simulink model "Servo_Model"  (R2019b)
settings: Solver=VariableStepAuto  StartTime=0.0  StopTime=100  RelTol=1e-3
values from neighbouring files (symbols this model uses):
  B = 0.1    [Servo_Param (1).m]    (also in servoParameters.m)
  Jd = 0.1    [Servo_Param (1).m]    (also in servoParameters.m = 1)
  Km = 1    [Servo_Param (1).m]    (also in servoParameters.m)
libraries: fl_lib x16, ee_lib x8, nesl_utility x8, fl_ps_legacy_lib x2, simulink x2
settings Model: Creator=covasanvictor  LastModifiedBy=covasanvictor
settings SolverCC: ZeroCrossAlgorithm=Adaptive
settings DataIOCC: Refine=100
settings DebuggingCC: MaskedZcDiagnostic=none  IgnoredZcDiagnostic=none
settings SFSimCC: CustomCodeUndefinedFunction=UseInterfaceOnly

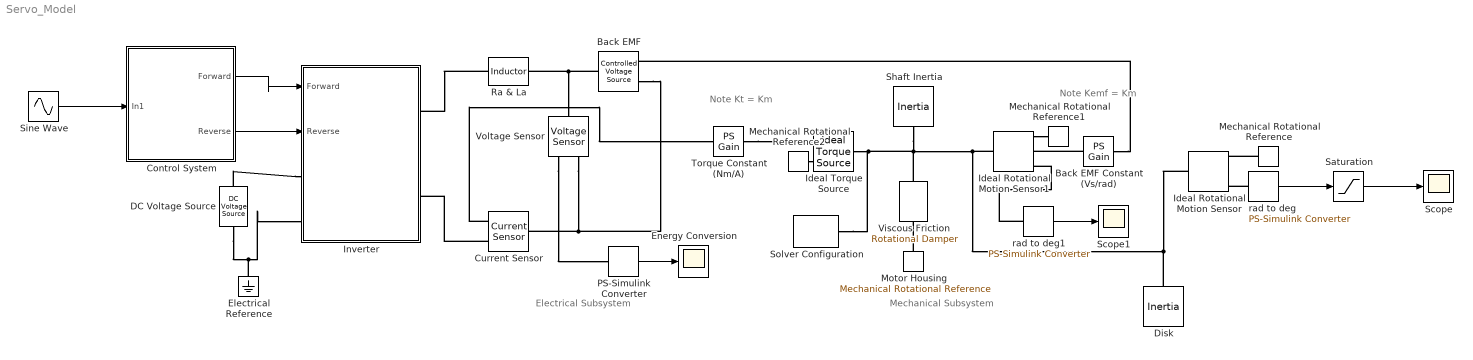
== system Servo_Model ==
  note: Mechanical
      | Subsystem
  note: Note
      | Kemf = Km
  note: Electrical
      | Subsystem
  note: Note
      | Kt = Km
  Back EMF : fl_lib/Electrical/Electrical Sources/Controlled Voltage Source
  Back EMF Constant (Vs/rad) : fl_ps_legacy_lib/Legacy Physical Signals/Functions/PS Gain  gain=Km
      settings: SourceProductName=Simscape
  Control System : Subsystem
  Current Sensor : fl_lib/Electrical/Electrical Sensors/Current Sensor
  DC Voltage Source : fl_lib/Electrical/Electrical Sources/DC Voltage Source  v0=6.2 V
  Disk : fl_lib/Mechanical/Rotational Elements/Inertia  inertia=Jd*21 kg*m^2  w_specify=off  w_priority=Low  w=0 rad/s  w_nominal_specify=off  w_nominal_unit=rad/s  w_nominal_value=1  t_specify=off  t_priority=None  t=0 N*m  t_nominal_specify=off  t_nominal_unit=N*m  t_nominal_value=1
  Electrical Reference : fl_lib/Electrical/Electrical Elements/Electrical Reference
  Energy Conversion : Scope
  Ideal Rotational Motion Sensor : fl_lib/Mechanical/Mechanical Sensors/Ideal Rotational Motion Sensor  offset=90 deg
  Ideal Rotational Motion Sensor1 : fl_lib/Mechanical/Mechanical Sensors/Ideal Rotational Motion Sensor  offset=90 deg
  Ideal Torque Source : fl_lib/Mechanical/Mechanical Sources/Ideal Torque Source
  Inverter : Subsystem
  Mechanical Rotational Reference : fl_lib/Mechanical/Rotational Elements/Mechanical Rotational Reference
  Mechanical Rotational Reference1 : fl_lib/Mechanical/Rotational Elements/Mechanical Rotational Reference
  Mechanical Rotational Reference2 : fl_lib/Mechanical/Rotational Elements/Mechanical Rotational Reference
  Motor Housing : fl_lib/Mechanical/Rotational Elements/Mechanical Rotational Reference
  PS-Simulink Converter : nesl_utility/PS-Simulink Converter  PhysicalDomain=network_engine_domain  SubClassName=ps_output  LeftPortType=input  RightPortType=output  PseudoPeriodic=off  Frequencies=[]  Unit=1  AffineConversion=off
  Ra & La : fl_lib/Electrical/Electrical Elements/Inductor  l=La H  r=Ra Ohm  g=0 1/Ohm  i_specify=off  i_priority=None  i=0 A  i_nominal_specify=off  i_nominal_unit=A  i_nominal_value=1  v_specify=off  v_priority=None  v=0 V  v_nominal_specify=off  v_nominal_unit=V  v_nominal_value=1  i_L_specify=off  i_L_priority=High  i_L=0 A  i_L_nominal_specify=off  i_L_nominal_unit=A  i_L_nominal_value=1
  Saturation : Saturate  UpperLimit=180  LowerLimit=-180
  Scope : Scope
  Scope1 : Scope
  Shaft Inertia : fl_lib/Mechanical/Rotational Elements/Inertia  inertia=J kg*m^2  w_specify=off  w_priority=High  w=0 rad/s  w_nominal_specify=off  w_nominal_unit=rad/s  w_nominal_value=1  t_specify=off  t_priority=None  t=0 N*m  t_nominal_specify=off  t_nominal_unit=N*m  t_nominal_value=1
  Sine Wave : Sin  Amplitude=70  Bias=100  Frequency=0.5  SampleTime=0
  Solver Configuration : nesl_utility/Solver Configuration  PhysicalDomain=network_engine_domain  SubClassName=solver  LeftPortType=input  RightPortType=generic  Tones=[]  Harmonics=[]  SimulateNoise=off  Profile=off  UseLocalSampling=off  EnableSwitchedLinearOptims=on  FrequencyDomain=off  UseCCode=off  RelTol=0.001  AbsTol=1e-06  MinStep=1e-09  ToWorkspace=off  RevertToSquareIcSolve=off  NumHomotopyIterations=100  PhasorMode=off  PhasorModeNumHarmonics=1  DoDC=off  ResidualTolerance=1e-9  UseLocalSolver=off  LocalSolverChoice=NE_BACKWARD_EULER_ADVANCER  LocalSolverSampleTime=.001  DoFixedCost=off  MaxNonlinIter=3  MaxModeIter=2  LinearAlgebra=Sparse  EquationFormulation=NE_TIME_EF  DelaysMemoryBudget=1024  AutomaticFiltering=on  FilteringTimeConstant=0.001  PartitionStorageMethod=AS_NEEDED  PartitionMemoryBudget=1024  PartitionMethod=FAST
  Torque Constant (Nm/A) : fl_ps_legacy_lib/Legacy Physical Signals/Functions/PS Gain  gain=Km
      settings: SourceProductName=Simscape
  Viscous Friction : fl_lib/Mechanical/Rotational Elements/Rotational Damper  D=B N*m/(rad/s)  w_specify=off  w_priority=None  w=0 rad/s  w_nominal_specify=off  w_nominal_unit=rad/s  w_nominal_value=1  t_specify=off  t_priority=None  t=0 N*m  t_nominal_specify=off  t_nominal_unit=N*m  t_nominal_value=1
  Voltage Sensor : fl_lib/Electrical/Electrical Sensors/Voltage Sensor
  rad to deg : nesl_utility/PS-Simulink Converter  PhysicalDomain=network_engine_domain  SubClassName=ps_output  LeftPortType=input  RightPortType=output  PseudoPeriodic=off  Frequencies=[]  Unit=deg  AffineConversion=off
  rad to deg1 : nesl_utility/PS-Simulink Converter  PhysicalDomain=network_engine_domain  SubClassName=ps_output  LeftPortType=input  RightPortType=output  PseudoPeriodic=off  Frequencies=[]  Unit=deg  AffineConversion=off
  wires:
  PS-Simulink Converter/1 -> Energy Conversion/1
  rad to deg1/1 -> Scope1/1
  rad to deg/1 -> Saturation/1
  Saturation/1 -> Scope/1
  Control System/1(Forward) -> Inverter/1(Forward)
  Control System/2(Reverse) -> Inverter/2(Reverse)
  Sine Wave/1 -> Control System/1(In1)
  connections:
  Solver Configuration/RConn1 -- Viscous Friction/RConn1 -- Ideal Rotational Motion Sensor/LConn1 -- Disk/LConn1 -- Ideal Rotational Motion Sensor1/LConn1 -- Shaft Inertia/LConn1 -- Ideal Torque Source/LConn1
  rad to deg/LConn1 -- Ideal Rotational Motion Sensor/RConn3
  Mechanical Rotational Reference/LConn1 -- Ideal Rotational Motion Sensor/RConn1
  Voltage Sensor/RConn2 -- Current Sensor/LConn1 -- Back EMF/RConn2
  Ra & La/RConn1 -- Back EMF/LConn1 -- Voltage Sensor/LConn1
  Current Sensor/RConn1 -- Torque Constant (Nm/A)/LConn1
  Mechanical Rotational Reference2/LConn1 -- Ideal Torque Source/RConn2
  Voltage Sensor/RConn1 -- PS-Simulink Converter/LConn1
  Torque Constant (Nm/A)/RConn1 -- Ideal Torque Source/RConn1
  Back EMF Constant (Vs/rad)/RConn1 -- Back EMF/RConn1
  Motor Housing/LConn1 -- Viscous Friction/LConn1
  Ideal Rotational Motion Sensor1/RConn1 -- Mechanical Rotational Reference1/LConn1
  Back EMF Constant (Vs/rad)/LConn1 -- Ideal Rotational Motion Sensor1/RConn2
  rad to deg1/LConn1 -- Ideal Rotational Motion Sensor1/RConn3
  DC Voltage Source/RConn1 -- Electrical Reference/LConn1 -- Inverter/LConn2
  Ra & La/LConn1 -- Inverter/RConn1
  DC Voltage Source/LConn1 -- Inverter/LConn1
  Current Sensor/RConn2 -- Inverter/RConn2

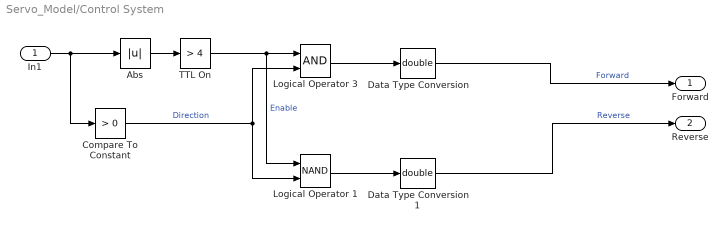
== system Servo_Model/Control System ==
  In1 : Inport
  Abs : Abs
  Compare To Constant : simulink/Logic and Bit Operations/Compare To Constant  relop=>  const=0  OutDataTypeStr=boolean  ZeroCross=off
  Data Type Conversion : DataTypeConversion  OutDataTypeStr=double
  Data Type Conversion1 : DataTypeConversion  OutDataTypeStr=double
  Logical Operator 1 : Logic  Operator=NAND  AllPortsSameDT=off  OutDataTypeStr=boolean
  Logical Operator 3 : Logic  AllPortsSameDT=off  OutDataTypeStr=boolean
  TTL On : simulink/Logic and Bit Operations/Compare To Constant  relop=>  const=4  OutDataTypeStr=boolean  ZeroCross=off
  Forward : Outport  VectorParamsAs1DForOutWhenUnconnected=off
  Reverse : Outport  Port=2  VectorParamsAs1DForOutWhenUnconnected=off
  wires:
  TTL On/1 -> Logical Operator 3/1, Logical Operator 1/1  "Enable"
  Compare To Constant/1 -> Logical Operator 1/2, Logical Operator 3/2  "Direction"
  Logical Operator 3/1 -> Data Type Conversion/1
  Data Type Conversion1/1 -> Reverse/1  "Reverse"
  Logical Operator 1/1 -> Data Type Conversion1/1
  Data Type Conversion/1 -> Forward/1  "Forward"
  In1/1 -> Abs/1, Compare To Constant/1
  Abs/1 -> TTL On/1

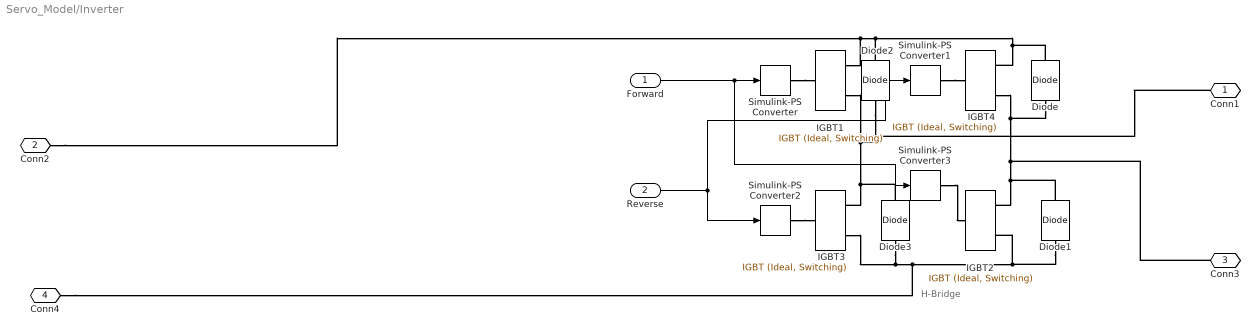
== system Servo_Model/Inverter ==
  note: H-Bridge
  Forward : Inport
  Reverse : Inport  Port=2
  Diode{,1..3} (4 alike) : ee_lib/Semiconductors & Converters/Diode  ModelType=ee.enum.diode.modelType.pwl  Vf=0.6 V  Ron=0.3 Ohm  Goff=1e-8 S  prmExp=ee.enum.diode.expParam.useTwo  I12=[.0137, .545] A  V12=[.6, .7] V  IS=1e-12 A  ec=1  I1=0.0137 A  V1=0.6 V  RS=0 Ohm  Tmeas=25 degC  N_series=1  N_parallel=1  Rz=0.3 Ohm  BV=inf V  C_param=ee.enum.diode.capParam.fixed  CJ=5 pF  CJ0=5 pF  VJ=1 V  Mgrad=0.5  Vvec=[.1, 10, 100] V  Cvec=[3.5, 1, .4] pF  FC=0.5  Q_param=ee.enum.diode.recoveryParam.off  iRM=-7.15 A  iF=4 A  didt=-750 A/us  trr_factor=3  trr=115 ns  Qrr=1500 s*uA  TT=50 ns  tau=100 ns  T_param=ee.enum.diode.temperatureParam.off  IS_T2=1.25e-7 A  I1_T2=0.245 A  V1_T2=0.5 V  Tmeas2=125 degC  EG_param=ee.enum.diode.egapParam.material_si  EG=1.11 eV  XTI_param=ee.enum.diode.xtiParam.pn  XTI=3  dBVdT=0 V/K  Tdevice=25 degC  i_specify=off  i_priority=None  i=0 A  i_nominal_specify=off  i_nominal_unit=A  i_nominal_value=1  v_specify=off  v_priority=None  v=0 V  v_nominal_specify=off  v_nominal_unit=V  v_nominal_value=1  i_capacitor_specify=off  i_capacitor_priority=None  i_capacitor=0 A  i_capacitor_nominal_specify=off  i_capacitor_nominal_unit=A  i_capacitor_nominal_value=1  v_capacitor_specify=off  v_capacitor_priority=None  v_capacitor=0 V  v_capacitor_nominal_specify=off  v_capacitor_nominal_unit=V  v_capacitor_nominal_value=1  power_dissipated_specify=off  power_dissipated_priority=None  power_dissipated=0 W  power_dissipated_nominal_specify=off  power_dissipated_nominal_unit=W  power_dissipated_nominal_value=1  thermal_network_parameterization=ee.enum.thermalNetworkTopology.cauer  Rth=[0, 10] K/W  Rth_Foster=[4, 6] K/W  thermal_mass_parameterization=ee.enum.thermalNetwork.timeconstant  thermal_mass=[0, 1] J/K  thermal_mass_Foster=[1.5, 3] J/K  thermal_time_constant=[0, 10] s  thermal_time_constant_Foster=[6, 18] s  thermal_mass_initial_temperatures=[25, 25] degC
      settings: SourceProductName=Simscape Electrical
  IGBT{1..4} (4 alike) : ee_lib/Semiconductors & Converters/IGBT (Ideal, Switching)  Vf=1 V  Ron=0.001 Ohm  Goff=1e-5 1/Ohm  Vth=0.5 V  diode_param=1  diode_Vf=0.8 V  diode_Ron=0.001 Ohm  diode_Goff=1e-5 1/Ohm  diode_C=5e-8 F  diode_iRM=-235 A  diode_iF=300 A  diode_idot=-50 A/us  diode_trr_param=1  diode_trr_factor=3  diode_trr=15 us  diode_Qrr=1.5e+3 s*uA  thermal_loss_option=2  Voff=300 V  Tau=1e-4 s  Tj=[298.15, 398.15] K  Iout_scalar=600 A  Eon_scalar=22.86e-3 J  Eoff_scalar=17.14e-3 J  Von_scalar=2.7 V  Iout_data=[0, 10, 50, 100, 200, 400, 600] A  Eon_data=[0, .29, 1.43, 2.86, 5.71, 13.14, 22.86; 0, .57, 2.63, 5.14, 10.29, 20.57, 30.29] * 1e-3 J  Eoff_data=[0, .21, 1.07, 2.14, 4.29, 9.86, 17.14; 0, .43, 1.97, 3.86, 7.71, 15.43, 22.71] * 1e-3 J  Von_data=[0, 1.1, 1.3, 1.45, 1.75, 2.25, 2.7; 0, 1, 1.15, 1.35, 1.7, 2.35, 3] V
      settings: SourceProductName=Simscape Electrical
  Simulink-PS Converter{,1..3} (4 alike) : nesl_utility/Simulink-PS Converter  PhysicalDomain=network_engine_domain  SubClassName=ps_input  LeftPortType=input  RightPortType=output  PseudoPeriodic=off  Frequencies=[]  NoiseDistribution=none  NoiseParameters=[]  Unit=1  AffineConversion=off  FilteringAndDerivatives=provide  SimscapeFilterOrder=1  InputFilterTimeConstant=0.001  UdotUserProvided=0
  Conn1 : PMIOPort  Side=Right
  Conn2 : PMIOPort  Port=2  Side=Left
  Conn3 : PMIOPort  Port=3  Side=Right
  Conn4 : PMIOPort  Port=4  Side=Left
  wires:
  Forward/1 -> Simulink-PS Converter3/1, Simulink-PS Converter/1
  Reverse/1 -> Simulink-PS Converter1/1, Simulink-PS Converter2/1
  connections:
  IGBT4/RConn2 -- Diode/LConn1 -- Conn3/RConn1 -- IGBT2/RConn1 -- Diode1/RConn1
  Conn2/RConn1 -- IGBT1/RConn1 -- Diode2/RConn1 -- Diode/RConn1 -- IGBT4/RConn1
  IGBT3/RConn2 -- Diode3/LConn1 -- Conn4/RConn1 -- IGBT2/RConn2 -- Diode1/LConn1
  IGBT1/RConn2 -- Conn1/RConn1 -- Diode2/LConn1 -- Diode3/RConn1 -- IGBT3/RConn1
  Simulink-PS Converter3/RConn1 -- IGBT2/LConn1
  Simulink-PS Converter2/RConn1 -- IGBT3/LConn1
  Simulink-PS Converter/RConn1 -- IGBT1/LConn1
  Simulink-PS Converter1/RConn1 -- IGBT4/LConn1
